simulink model "kapitsa_pendulum"  (R2023a)
settings: Solver=FixedStepAuto  StartTime=0.0  StopTime=500  FixedStep=0.01  MaxStep=0.05  RelTol=1e-3
values from neighbouring files (symbols this model uses):
  I = m * l^2    [mask.m]
undefined symbols (not defined in the file or in its folder): Amplitude, nu, startAngel
libraries: simulink_extras x2
settings Model: Creator=tanov  LastModifiedBy=tanov
settings DataIOCC: ReturnWorkspaceOutputs=off

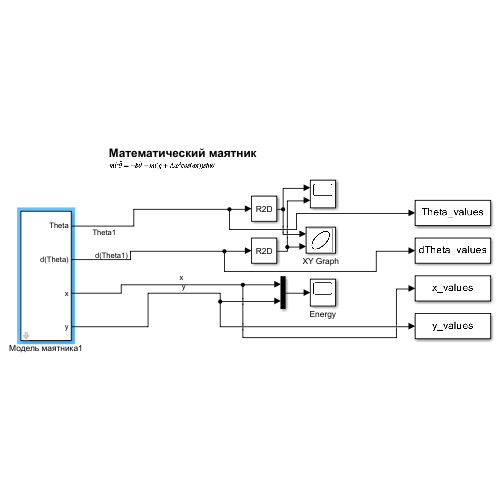
[thumbnail: Simulink's stored preview of the top-level diagram]
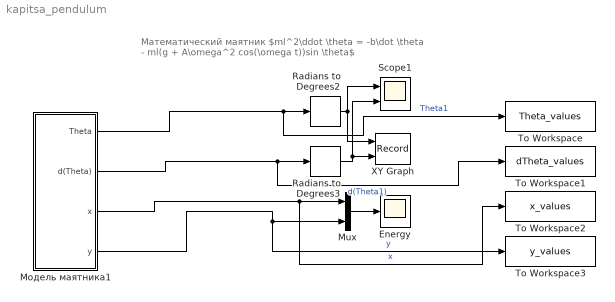
== system kapitsa_pendulum ==
  note: Математический маятник
      | $ml^2\ddot \theta = -b\dot \theta - ml(g + A\omega^2 cos(\omega t))sin \theta$
  Energy : Scope
  Mux : Mux  Inputs=2
  Radians to Degrees2 : simulink_extras/Transformations/Radians to Degrees
  Radians to Degrees3 : simulink_extras/Transformations/Radians to Degrees
  Scope1 : Scope  NumInputPorts=2
  To Workspace : ToWorkspace  VariableName=Theta_values  SampleTime=-1
      settings: Save2DSignal=2-D array (concatenate along first dimension)
  To Workspace1 : ToWorkspace  VariableName=dTheta_values  SampleTime=-1
      settings: Save2DSignal=2-D array (concatenate along first dimension)
  To Workspace2 : ToWorkspace  VariableName=x_values  SampleTime=-1
      settings: Save2DSignal=2-D array (concatenate along first dimension)
  To Workspace3 : ToWorkspace  VariableName=y_values  SampleTime=-1
      settings: Save2DSignal=2-D array (concatenate along first dimension)
  XY Graph : Record  FileSettingsInternal="{\"entries\":[{\"content\":{\"excelSettings\":{\"content\":{},\"type\":\"Streamout.ExcelSettings\"}},\"type\":\"Streamout.FileSettingStorage\",\"uuid\":\"5cae85d7-e527-43ed-8075-8f85d7bce30c\"}],\"packageUris\":[\"http://schema.mathworks.com/mf0/streamout_blocks/R2020a\"],\"version\":\"1.0\"}"  Layout=[1 1]  SignalsInternal="{\"entries\":[{\"content\":{\"signals\":[{\"content\":{\"blockPath\":[\"kapitsa_pendulum/XY Graph\"],\"dimensions\":[1],\"domain\":\"kapitsa_pendulum/XY Graph\",\"lineColor\":\"#a2142f\",\"plots\":[1],\"port\":1,\"sid\":[\"\"],\"signalID\":6251,\"signalName\":\"Radians\\nto Degrees2\"},\"type\":\"RecordBlkView.Signal\",\"uuid\":\"2de76a88-1e43-4704-b5c1-454f01a73b99\"},{\"content\":{\"blockPath\":[\"kapitsa_pendulum/XY Graph\"],\"dimensions\":[1],\"domain\":\"kapitsa_pendulum/XY Graph\",\"lineColor\":\"#139fff\",\"plots\":[1],\"port\":2,\"sid\":[\"\"],\"signalID\":6255,\"signalName\":\"Radians\\nto Degrees3\"},\"type\":\"RecordBlkView.Signal\",\"uuid\":\"e4b7c61f-ea3d-4700-a610-1261e53e623f\"}]},\"type\":\"RecordBlkView.InputSignals\",\"uuid\":\"f735c356-b3cc-4235-b729-de321f8efc1b\"}],\"packageUris\":[\"http://schema.mathworks.com/mf0/streamout_blocks/R2020a\"],\"version\":\"1.0\"}"  VisualizationBindings="{\"xyplotplugin\":{\"info\":[{\"series\":[{\"bindingParametersList\":[{\"parameter\":\"X-Axis\",\"signalID\":6251,\"signalName\":\"Radians\\nto Degrees2\"},{\"parameter\":\"Y-Axis\",\"signalID\":6255,\"signalName\":\"Radians\\nto Degrees3\"}],\"seriesID\":14889}],\"subplotID\":1}]}}"  CompatibilityTag=XY
  Модель маятника1 : Subsystem  mask{m=1, L=9.8, g=9.8, startDegree=startAngel, b=0.01}
      mask prompts: m "Масса"; L "Длина подвеса"; g "Угловая скорость"; startDegree "Начальный угол"; b "Коэффициент затухания"
  wires:
  Модель маятника1/2(d(Theta)) -> To Workspace1/1, Radians to Degrees3/1  "d(Theta1)"
  Модель маятника1/1(Theta) -> To Workspace/1, Radians to Degrees2/1  "Theta1"
  Radians to Degrees3/1 -> XY Graph/2, Scope1/2
  Radians to Degrees2/1 -> XY Graph/1, Scope1/1
  Модель маятника1/4(y) -> To Workspace3/1, Mux/2  "y"
  Модель маятника1/3(x) -> To Workspace2/1, Mux/1  "x"
  Mux/1 -> Energy/1

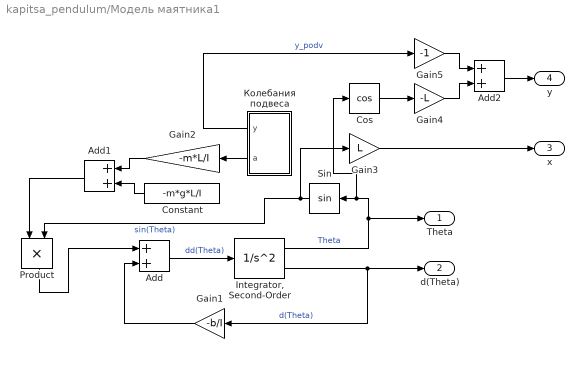
== system kapitsa_pendulum/Модель маятника1 ==
  Add : Sum
  Add1 : Sum
  Add2 : Sum
  Constant : Constant  Value=-m*g*L/I
  Cos : Trigonometry  Operator=cos
  Gain1 : Gain  Gain=-b/I
  Gain2 : Gain  Gain=-m*L/I
  Gain3 : Gain  Gain=L
  Gain4 : Gain  Gain=-L
  Gain5 : Gain  Gain=-1
  "Integrator, Second-Order" : SecondOrderIntegrator  ICX=deg2rad(startDegree)  ICDXDT=0
  Product : Product
  Sin : Trigonometry
  Колебания подвеса : Subsystem  mask{A=Amplitude, nu=nu}
      mask prompts: A "Амплитуда колебаний"; nu "Частота колебаний"
  Theta : Outport
  d(Theta) : Outport  Port=2
  x : Outport  Port=3
  y : Outport  Port=4
  wires:
  Sin/1 -> Product/2, Gain3/1  "sin(Theta)"
  "Integrator, Second-Order"/1 -> Theta/1, Cos/1, Sin/1  "Theta"
  "Integrator, Second-Order"/2 -> Gain1/1, d(Theta)/1  "d(Theta)"
  Add/1 -> "Integrator, Second-Order"/1  "dd(Theta)"
  Gain1/1 -> Add/2
  Колебания подвеса/2(a) -> Gain2/1
  Gain2/1 -> Add1/1
  Gain3/1 -> x/1
  Cos/1 -> Gain4/1
  Колебания подвеса/1(y) -> Gain5/1  "y_podv"
  Gain5/1 -> Add2/1
  Gain4/1 -> Add2/2
  Add2/1 -> y/1
  Constant/1 -> Add1/2
  Add1/1 -> Product/1
  Product/1 -> Add/1

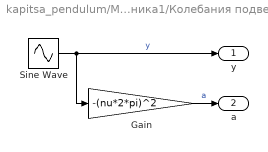
== system kapitsa_pendulum/Модель маятника1/Колебания подвеса ==
  Gain : Gain  Gain=-(nu*2*pi)^2
  Sine Wave : Sin  Amplitude=A  Frequency=nu*2*pi  SampleTime=0
  y : Outport
  a : Outport  Port=2
  wires:
  Gain/1 -> a/1  "a"
  Sine Wave/1 -> y/1, Gain/1  "y"
